simulink model "simulador_trayectorias_AN5"  (R2024a)
settings: Solver=FixedStepAuto  StartTime=0.0  StopTime=Tfinal  FixedStep=0.1  RelTol=1e-3
undefined symbols (not defined in the file or in its folder): fr5_ik, visualizar_robot_simulink
settings Model: Creator=angel  LastModifiedBy=angel

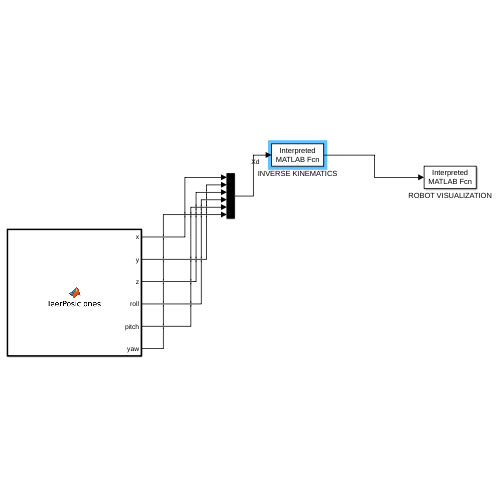
[thumbnail: Simulink's stored preview of the top-level diagram]
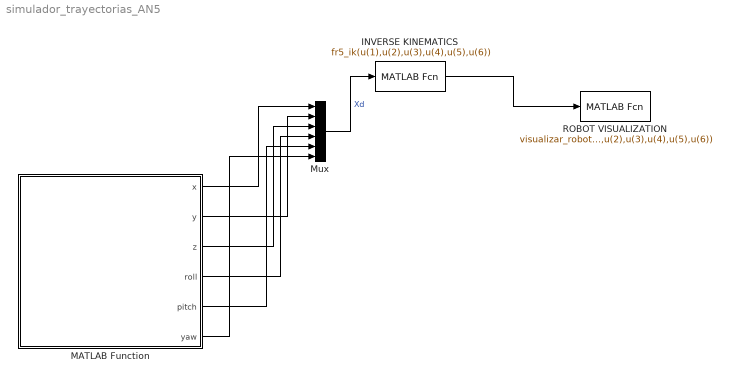
== system simulador_trayectorias_AN5 ==
  INVERSE KINEMATICS : MATLABFcn  MATLABFcn=fr5_ik(u(1),u(2),u(3),u(4),u(5),u(6))  OutputDimensions=6
  MATLAB Function : MATLAB Function  TreatAsAtomicUnit=on
  Mux : Mux  Inputs=6
  ROBOT VISUALIZATION : MATLABFcn  MATLABFcn=visualizar_robot_simulink(u(1),u(2),u(3),u(4),u(5),u(6))  OutputDimensions=0
  wires:
  Mux/1 -> INVERSE KINEMATICS/1  "Xd"
  INVERSE KINEMATICS/1 -> ROBOT VISUALIZATION/1
  MATLAB Function/1(x) -> Mux/1
  MATLAB Function/2(y) -> Mux/2
  MATLAB Function/3(z) -> Mux/3
  MATLAB Function/4(roll) -> Mux/4
  MATLAB Function/5(pitch) -> Mux/5
  MATLAB Function/6(yaw) -> Mux/6

== matlab function simulador_trayectorias_AN5/MATLAB Function ==
  data: x output; y output; z output; roll output; pitch output; yaw output
function [x, y, z, roll, pitch, yaw] = leerPosiciones()
    % Variables persistentes para mantener el estado entre iteraciones
    persistent posiciones rotaciones indice n_puntos;
    
    % Solo inicializamos la primera vez
    if isempty(posiciones)
        % Nombre del archivo de posiciones
        archivo_salida_txt = 'desired_positions.txt';
        
        % Abrir el archivo
        fileID = fopen(archivo_salida_txt, 'r');
        if fileID == -1
            error('No se pudo abrir el archivo de posiciones.');
        end
        
        % Leer y descartar la primera línea (cabecera)
        fgetl(fileID);
        
        % Leer todas las filas restantes con al menos 8 columnas y desechar la séptima y octava
        data = fscanf(fileID, '%f,%f,%f,%f,%f,%f,%*f,%*f', [6, Inf])';
        
        % Cerrar el archivo
        fclose(fileID);
        
        % Separar posiciones y rotaciones de los datos
        posiciones = data(:, 1:3);   % Columnas 1, 2, 3 son X, Y, Z
        rotaciones = data(:, 4:6);     % Columnas 4, 5, 6 son Roll, Pitch, Yaw
        n_puntos = size(posiciones, 1);  % Número total de puntos
        indice = 1;  % Iniciamos desde el primer punto
    end

    % Controlamos el índice para no sobrepasar el número total de puntos
    if indice > n_puntos
        % Si se han recorrido todos los puntos, se mantiene el índice en el último
        indice = n_puntos;
    end

    % Extraer la posición y rotación actuales
    x = posiciones(indice, 1);
    y = posiciones(indice, 2);
    z = posiciones(indice, 3);
    roll = rotaciones(indice, 1);
    pitch = rotaciones(indice, 2);
    yaw = rotaciones(indice, 3);

    % Avanzar al siguiente punto solo si no estamos en el último punto
    if indice < n_puntos
        indice = indice + 1;
    end
end
